simulink model "modelo"  (R2021b)
settings: Solver=VariableStepAuto  StartTime=0.0  StopTime=5  RelTol=1e-3
values from neighbouring files (symbols this model uses):
  h = 0.005    [script.m]
  L = dlqr(phi,gama,Q1,Q2)    [script.m]
  qi = [0;pi]    [script.m]
  qi1 = [0;pi/7]    [script.m]
settings Model: Creator=Dylan  LastModifiedBy=Dylan

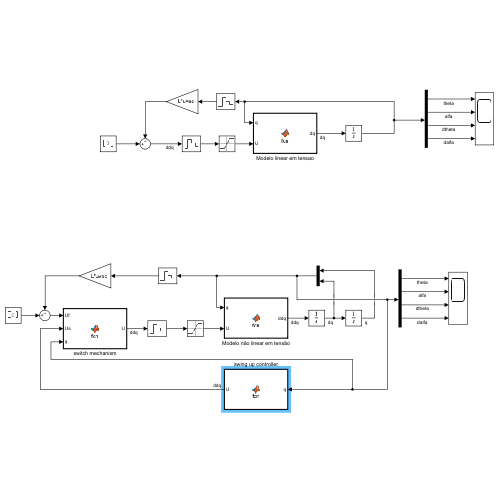
[thumbnail: Simulink's stored preview of the top-level diagram]
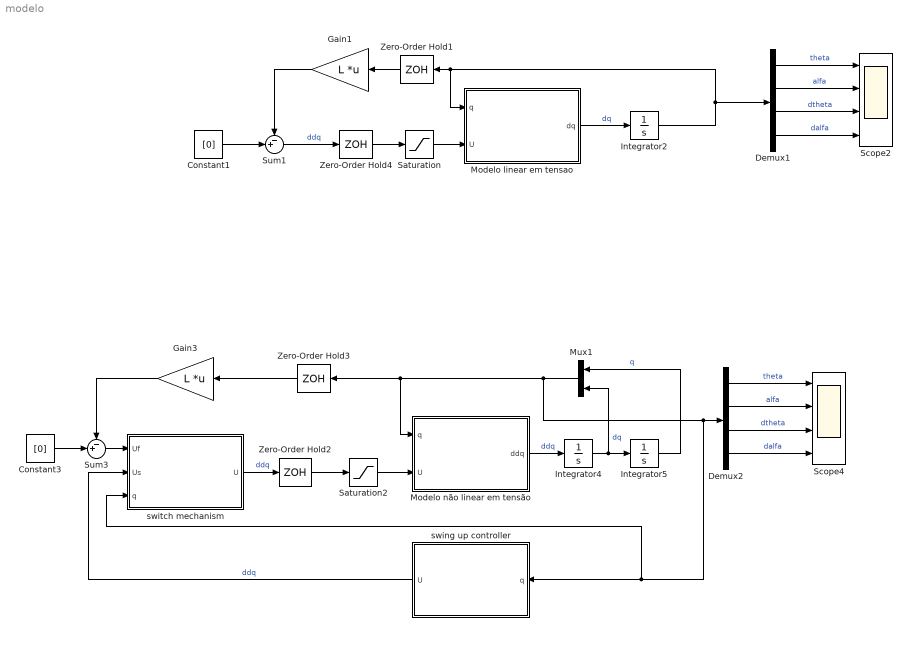
== system modelo ==
  Constant1 : Constant  Value=[0]
  Constant3 : Constant  Value=[0]
  Demux1 : Demux
  Demux2 : Demux
  Gain1 : Gain  Gain=L  Multiplication=Matrix(K*u) (u vector)
  Gain3 : Gain  Gain=L  Multiplication=Matrix(K*u) (u vector)
  Integrator2 : Integrator  InitialCondition=[qi1;0;0]
  Integrator4 : Integrator  InitialCondition=[0;0]
  Integrator5 : Integrator  InitialCondition=[qi]
  Modelo linear em tensao : MATLAB Function  TreatAsAtomicUnit=on
  Modelo não linear em tensão : MATLAB Function  TreatAsAtomicUnit=on
  Mux1 : Mux  Inputs=2
  Saturation : Saturate  UpperLimit=6  LowerLimit=-6
  Saturation2 : Saturate  UpperLimit=6  LowerLimit=-6
  Scope2 : Scope  NumInputPorts=4
  Scope4 : Scope  NumInputPorts=4
  Sum1 : Sum  Inputs=-+|
  Sum3 : Sum  Inputs=-+|
  Zero-Order Hold{1..4} (4 alike) : ZeroOrderHold  SampleTime=h
  swing up controller : MATLAB Function  TreatAsAtomicUnit=on
  switch mechanism : MATLAB Function  TreatAsAtomicUnit=on
  wires:
  Zero-Order Hold1/1 -> Gain1/1
  Constant1/1 -> Sum1/2
  Modelo linear em tensao/1(dq) -> Integrator2/1  "dq"
  Integrator2/1 -> Zero-Order Hold1/1, Modelo linear em tensao/1(q), Demux1/1
  Demux1/1 -> Scope2/1  "theta"
  Zero-Order Hold3/1 -> Gain3/1
  Gain3/1 -> Sum3/1
  Modelo não linear em tensão/1(ddq) -> Integrator4/1  "ddq"
  Constant3/1 -> Sum3/2
  Integrator4/1 -> Mux1/2, Integrator5/1  "dq"
  Integrator5/1 -> Mux1/1  "q"
  Saturation/1 -> Modelo linear em tensao/2(U)
  Demux1/2 -> Scope2/2  "alfa"
  Demux1/3 -> Scope2/3  "dtheta"
  Demux1/4 -> Scope2/4  "dalfa"
  Demux2/4 -> Scope4/4  "dalfa"
  Demux2/2 -> Scope4/2  "alfa"
  Demux2/3 -> Scope4/3  "dtheta"
  Demux2/1 -> Scope4/1  "theta"
  Mux1/1 -> switch mechanism/3(q), swing up controller/1(q), Demux2/1, Modelo não linear em tensão/1(q), Zero-Order Hold3/1
  Sum3/1 -> switch mechanism/1(Uf)
  swing up controller/1(U) -> switch mechanism/2(Us)  "ddq"
  Gain1/1 -> Sum1/1
  Sum1/1 -> Zero-Order Hold4/1  "ddq"
  Zero-Order Hold4/1 -> Saturation/1
  Zero-Order Hold2/1 -> Saturation2/1
  Saturation2/1 -> Modelo não linear em tensão/2(U)
  switch mechanism/1(U) -> Zero-Order Hold2/1  "ddq"

== matlab function modelo/Modelo linear em tensao ==
  data: q input; dq output; U input
function dq  = fcn(q,U)
%parametros motor
Rm = 2.6;
Km = 0.00767;
Kg = 70;
mp = 0.126;
Lp = 0.33;
lp = Lp/2;
r = 0.22;
Jb = 0.0044;
g = 9.8;

% modelo linerar em tensão
A = [0 0 1 0
0 0 0 1
0 -(mp*r*g)/Jb -((Km*Kg)^2)/(Rm*Jb) 0
0 g*(Jb+(mp*(r^2)))/(lp*Jb) r*((Km*Kg)^2)/(Rm*Jb*lp) 0
];

B = [0;0;(Km*Kg)/(Rm*Jb);-r*(Km*Kg)/(Rm*lp*Jb)];

dq = A*q+B.*U;
end

== matlab function modelo/swing up controller ==
  data: q input; U output
function U  = fcn(q)
%parametros motor
Rm = 2.6;
Km = 0.00767;
Kg = 70;
mp = 0.126;
Lp = 0.33;
lp = Lp/2;
r = 0.22;
Jb = 0.0044;
g = 9.8;
n= 0.4;
k =15;

theta=q(1);
alfa=q(2);
dtheta=q(3);
dalfa=q(4);

w0 = sqrt(mp*g*Lp/Jb);
E=mp*g*lp*(0.5*(dalfa/w0)^2+cos(alfa)-1);

u =  k*(E-0.1);
if u> n*g
    u = n*g;
elseif u<-n*g 
    u = -n*g;
end

U = u*sign(dalfa*cos(alfa));
end

== matlab function modelo/switch mechanism ==
  data: Uf input; Us input; q input; U output
function U  = fcn(Uf,Us,q)
theta=q(1);
alfa=q(2);
dtheta=q(3);
dalfa=q(4);

if abs(alfa)<deg2rad(30)
    U = Uf;
else
    U = Us;
end
end

== matlab function modelo/Modelo não linear em tensão ==
  data: q input; ddq output; U input
function ddq  = fcn(q,U)
%parametros motor
Rm = 2.6;
Km = 0.00767;
Kg = 70;
mp = 0.126;
Lp = 0.33;
lp = Lp/2;
r = 0.22;
Jb = 0.0044;
g = 9.8;

theta=q(1);
alfa=q(2);
dtheta=q(3);
dalfa=q(4);

a = Jb + mp*r^2;
b = mp*r*lp*cos(alfa);
c = mp*lp*r*cos(alfa);
d = mp*lp^2;
M = [a b;c d];

Vb = U;
Tb = (Kg*Km)*(Vb-Kg*Km*dtheta)/Rm;

a = -mp*r*dalfa^2*lp*sin(alfa);
b = -mp*g*lp*sin(alfa); 
H = [a;b];

ddq = inv(M)*([Tb;0]-H);
end
